simulink model "VisionModel_v6"  (Simulink 7.6)
settings: Solver=FixedStepDiscrete  StartTime=0.0  StopTime=0  RelTol=1e-3
values from neighbouring files (symbols this model uses):
  Iter_Segment_Thresh = 60    [VisionConstants.m]
  Scale_Down_B = 1    [VisionConstants.m]
  Scale_Down_G = 1    [VisionConstants.m]
  Scale_Down_H = 1    [VisionConstants.m]
  Scale_Down_R = 1    [VisionConstants.m]
  Scale_Down_S = 1    [VisionConstants.m]
  Scale_Down_V = 5    [VisionConstants.m]
  Scale_Forward_B = 0    [VisionConstants.m]
  Scale_Forward_G = 1    [VisionConstants.m]
  Scale_Forward_H = 1    [VisionConstants.m]
  Scale_Forward_R = 0    [VisionConstants.m]
  Scale_Forward_S = 1    [VisionConstants.m]
  Scale_Forward_V = 5    [VisionConstants.m]
undefined symbols (not defined in the file or in its folder): Rec, SDTV
libraries: vipconversions x4
settings Model: Creator=Administrator  LastModifiedBy=auvt
settings OptimizationCC: OptimizeModelRefInitCode=on
settings RTWCC: SystemTargetFile=ert.tlc  GenCodeOnly=on  TemplateMakefile=ert_default_tmf  PostCodeGenCommand=packNGo(buildInfo, {'packType' 'flat'})  Description=Real-Time Workshop Embedded Coder  GenerateReport=on  ProcessScript=ert_make_rtw_hook  IncludeHyperlinkInReport=on  LaunchReport=on  TargetLang=C++
settings CodeAppCC: IgnoreCustomStorageClasses=off
settings ERTTargetCC: MultiwordLength=2048  GenerateSampleERTMain=on  IncludeMdlTerminateFcn=off  ERTCustomFileTemplate=example_file_process.tlc  ConvertIfToSwitch=off

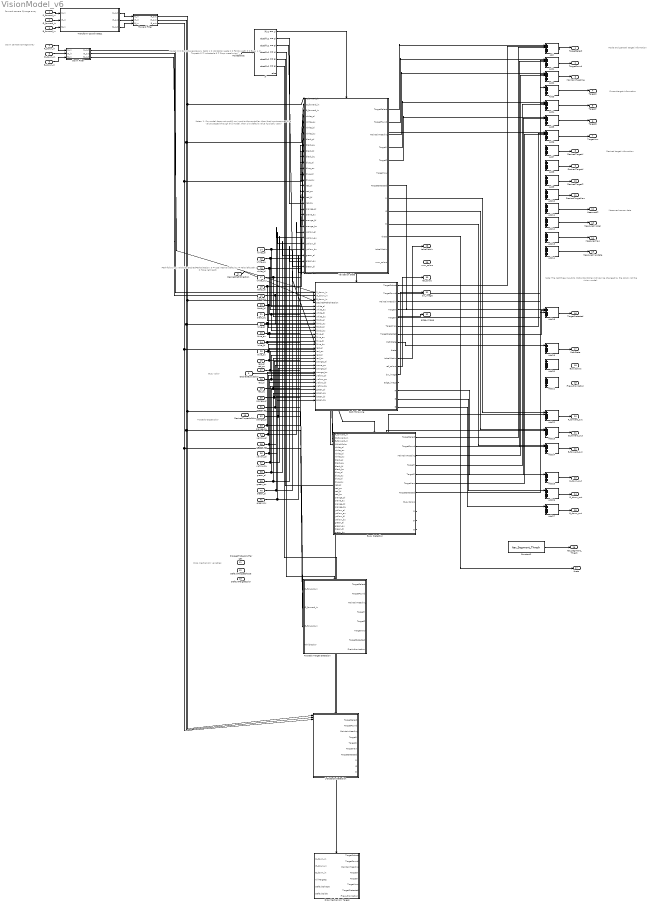
== system VisionModel_v6 ==
  note: Current target information
  note: Desired target information
  note: Measured sensor data
  note: Mode and general target information
  note: Forward camera QImage array
  note: Modes:
      | 0 = Do not execute any tasks
      | 1 = Validation gate
      | 2 = Follow path
      | 3 = Buoy
      | 4 = Torpedo
      | 5 = L-obstacle
      | 6 = Drop mecahnism
  note: Path-following variables
      | DesiredPathDirection:
      | 0 = Use internal default
      | 1 = Take left path
      | 2 = Take right path
  note: Buoy color
  note: Torpedo target color
  note: Drop mechanism variables
  note: Down camera QImage array
  note: Notes:
      | 1. If a model does not modify an input to the controller,
      | then that input assumes 1) a value passed through this
      | model, then 2) a default value (typically zero)
  note: Note: The last three inputs to MotionController.mdl
      | can be changed by the script, not the vision model.
  R_forward_in : Inport  PortDimensions=Forward_Camera_Dimensions
  G_forward_in : Inport  Port=2  PortDimensions=Forward_Camera_Dimensions
  B_forward_in : Inport  Port=3  PortDimensions=Forward_Camera_Dimensions
  R_down_in : Inport  Port=4  PortDimensions=Down_Camera_Dimensions
  G_down_in : Inport  Port=5  PortDimensions=Down_Camera_Dimensions
  B_down_in : Inport  Port=6  PortDimensions=Down_Camera_Dimensions
  ModeSelect : Inport  Port=7
  DesiredPathDirection : Inport  Port=8
  DesiredBuoyColor : Inport  Port=9
  DesiredTorpedoColor : Inport  Port=10
  ProceedToSecondTarget : Inport  Port=11
  DefaultTargetShape : Inport  Port=12
  DefaultTargetColor : Inport  Port=13
  white_al : Inport  Port=14
  white_au : Inport  Port=15
  white_bl : Inport  Port=16
  white_bu : Inport  Port=17
  black_al : Inport  Port=18
  black_au : Inport  Port=19
  black_bl : Inport  Port=20
  black_bu : Inport  Port=21
  blue_al : Inport  Port=22
  blue_au : Inport  Port=23
  blue_bl : Inport  Port=24
  blue_bu : Inport  Port=25
  red_al : Inport  Port=26
  red_au : Inport  Port=27
  red_bl : Inport  Port=28
  red_bu : Inport  Port=29
  orange_al : Inport  Port=30
  orane_au : Inport  Port=31
  orange_bl : Inport  Port=32
  orange_bu : Inport  Port=33
  yellow_al : Inport  Port=34
  yellow_au : Inport  Port=35
  yellow_bl : Inport  Port=36
  yellow_bu : Inport  Port=37
  green_al : Inport  Port=38
  green_au : Inport  Port=39
  breen_bl : Inport  Port=40
  green_bu : Inport  Port=41
  Add{,1..14,18..27} (25 alike) : Sum  Inputs=++++++
  Buoy Detection : Subsystem  TreatAsAtomicUnit=on
  Constant2 : Constant  Value=Iter_Segment_Thresh  SampleTime=-1
  Down Filter : Subsystem
  Drop Mechanism Target : Subsystem  TreatAsAtomicUnit=on
  Forward Filter : Subsystem
  If : If  IfExpression=u1 == 1  ElseIfExpressions=u1 == 2, u1 == 3, u1 == 4, u1 == 5, u1 == 6
  L-Obstacle Detection : Subsystem  TreatAsAtomicUnit=on
  Path Following : Subsystem  TreatAsAtomicUnit=on
  Torpedo Target Detection : Subsystem  TreatAsAtomicUnit=on
  Transform Coordinates1 : Stateflow chart  TreatAsAtomicUnit=on  SystemSampleTime=[1/30 0]
  Validation Gate : Subsystem  TreatAsAtomicUnit=on
  TargetSelect : Outport  OutDataTypeStr=double
  TargetFound : Outport  Port=2  OutDataTypeStr=double
  MaintainHeading : Outport  Port=3  OutDataTypeStr=double
  TargetX : Outport  Port=4  OutDataTypeStr=double
  TargetY : Outport  Port=5  OutDataTypeStr=double
  TargetZ : Outport  Port=6  OutDataTypeStr=double
  TargetYaw : Outport  Port=7  OutDataTypeStr=double
  DesiredTargetX : Outport  Port=8  OutDataTypeStr=double
  DesiredTargetY : Outport  Port=9  OutDataTypeStr=double
  DesiredTargetZ : Outport  Port=10  OutDataTypeStr=double
  DesiredTargetYaw : Outport  Port=11  OutDataTypeStr=double
  MeasuredZ : Outport  Port=12  OutDataTypeStr=double
  MeasuredYAccel : Outport  Port=13  OutDataTypeStr=double
  MeasuredYaw : Outport  Port=14  OutDataTypeStr=double
  MeasuredYawRate : Outport  Port=15  OutDataTypeStr=double
  TargetDetected : Outport  Port=16  OutDataTypeStr=double
  PathState : Outport  Port=17  OutDataTypeStr=double
  BuoyColors : Outport  Port=18  OutDataTypeStr=double
  FireAuthorization : Outport  Port=19  OutDataTypeStr=double
  R_forward_out : Outport  Port=20  OutDataTypeStr=double
  G_forward_out : Outport  Port=21  OutDataTypeStr=double
  B_forward_out : Outport  Port=22  OutDataTypeStr=double
  R_down_out : Outport  Port=23  OutDataTypeStr=double
  G_down_out : Outport  Port=24  OutDataTypeStr=double
  B_down_out : Outport  Port=25  OutDataTypeStr=double
  Iter_Segment_Thresh : Outport  Port=26  OutDataTypeStr=double
  theta : Outport  Port=27  OutDataTypeStr=double
  LabelMatrix : Outport  Port=28
  num_colors : Outport  Port=29
  ref_colors : Outport  Port=30
  bw_image : Outport  Port=31
  edge_image : Outport  Port=32
  wires:
  ModeSelect/1 -> If/1
  If/2 -> Path Following/Action
  If/3 -> Buoy Detection/Action
  If/1 -> Validation Gate/Action
  If/4 -> Torpedo Target Detection/Action
  If/5 -> L-Obstacle Detection/Action
  If/6 -> Drop Mechanism Target/Action
  DesiredBuoyColor/1 -> Buoy Detection/4(WhichColor)
  Down Filter/1(R_out) -> Path Following/1(R_down_in)
  Down Filter/2(G_out) -> Path Following/2(G_down_in)
  Down Filter/3(B_out) -> Path Following/3(B_down_in)
  Add/1 -> TargetSelect/1
  Add1/1 -> TargetFound/1
  Add2/1 -> MaintainHeading/1
  Add3/1 -> TargetX/1
  Add4/1 -> TargetY/1
  Add5/1 -> TargetZ/1
  Add6/1 -> TargetYaw/1
  Add7/1 -> DesiredTargetX/1
  Add8/1 -> DesiredTargetY/1
  Add9/1 -> DesiredTargetZ/1
  Add10/1 -> DesiredTargetYaw/1
  Add11/1 -> MeasuredZ/1
  Add12/1 -> MeasuredYAccel/1
  Add13/1 -> MeasuredYaw/1
  Add14/1 -> MeasuredYawRate/1
  Forward Filter/2(G_out) -> Validation Gate/2(G_forward_in), Buoy Detection/2(G_forward_in), Torpedo Target Detection/2(G_forward_in), L-Obstacle Detection/2(G_forward_in)
  Forward Filter/3(B_out) -> Validation Gate/3(B_forward_in), Buoy Detection/3(B_forward_in), Torpedo Target Detection/3(B_forward_in), L-Obstacle Detection/3(B_forward_in)
  Forward Filter/1(R_out) -> Validation Gate/1(R_forward_in), Buoy Detection/1(R_forward_in), Torpedo Target Detection/1(R_forward_in), L-Obstacle Detection/1(R_forward_in)
  G_down_in/1 -> Down Filter/2(G_in)
  R_down_in/1 -> Down Filter/1(R_in)
  B_down_in/1 -> Down Filter/3(B_in)
  Validation Gate/5(TargetZ) -> Add5/1
  Validation Gate/4(TargetY) -> Add4/1
  Validation Gate/1(TargetSelect) -> Add/1
  Validation Gate/2(TargetFound) -> Add1/1
  Validation Gate/3(MaintainHeading) -> Add2/1
  Validation Gate/6(TargetYaw) -> Add6/1
  Validation Gate/7(TargetDetected) -> Add18/1
  Add18/1 -> TargetDetected/1
  Constant2/1 -> Iter_Segment_Thresh/1
  Validation Gate/11(theta) -> theta/1
  G_forward_in/1 -> Transform Coordinates1/2(G_in)
  R_forward_in/1 -> Transform Coordinates1/1(R_in)
  B_forward_in/1 -> Transform Coordinates1/3(B_in)
  Transform Coordinates1/1(R_out) -> Forward Filter/1(R_in)
  Transform Coordinates1/2(G_out) -> Forward Filter/2(G_in)
  Transform Coordinates1/3(B_out) -> Forward Filter/3(B_in)
  Path Following/10(LabelMatrix) -> LabelMatrix/1
  ? -> num_colors/1
  Path Following/11(ref_colors) -> ref_colors/1
  Path Following/12(bw_image) -> bw_image/1
  Path Following/13(edge_image) -> edge_image/1
  Path Following/1(TargetSelect) -> Add/2
  Path Following/2(TargetFound) -> Add1/2
  Path Following/3(MaintainHeading) -> Add2/2
  Path Following/4(TargetX) -> Add3/1
  Path Following/5(TargetY) -> Add4/2
  Path Following/6(TargetYaw) -> Add6/2
  Path Following/7(TargetDetected) -> Add18/2
  Path Following/8(PathState) -> Add19/1
  Add19/1 -> PathState/1
  DesiredPathDirection/1 -> Path Following/4(DesiredPathDirection)
  Add22/1 -> R_forward_out/1
  Add23/1 -> G_forward_out/1
  Add24/1 -> B_forward_out/1
  Validation Gate/8(R) -> Add22/1
  Validation Gate/9(G) -> Add23/1
  Validation Gate/10(B) -> Add24/1
  Path Following/14(R) -> Add25/1
  Path Following/15(G) -> Add26/1
  Path Following/16(B) -> Add27/1
  Add25/1 -> R_down_out/1
  Add26/1 -> G_down_out/1
  Add27/1 -> B_down_out/1
  Buoy Detection/9(R) -> Add22/2
  Buoy Detection/10(G) -> Add23/2
  Buoy Detection/11(B) -> Add24/2
  Buoy Detection/1(TargetSelect) -> Add/3
  Buoy Detection/2(TargetFound) -> Add1/3
  Buoy Detection/3(MaintainHeading) -> Add2/3
  Buoy Detection/4(TargetY) -> Add4/3
  Buoy Detection/5(TargetZ) -> Add5/2
  Buoy Detection/6(TargetYaw) -> Add6/3
  Buoy Detection/7(TargetDetected) -> Add18/3
  white_al/1 -> Validation Gate/4(white_al), Path Following/5(white_al)
  white_au/1 -> Validation Gate/5(white_au), Path Following/6(white_au)
  white_bl/1 -> Validation Gate/6(white_bl), Path Following/7(white_bl)
  white_bu/1 -> Validation Gate/7(white_bu), Path Following/8(white_bu)
  black_al/1 -> Validation Gate/8(black_al), Path Following/9(black_al)
  black_au/1 -> Validation Gate/9(black_au), Path Following/10(black_au)
  black_bl/1 -> Validation Gate/10(black_bl), Path Following/11(black_bl)
  black_bu/1 -> Validation Gate/11(black_bu), Path Following/12(black_bu)
  blue_al/1 -> Validation Gate/12(blue_al), Path Following/13(blue_al)
  blue_au/1 -> Validation Gate/13(blue_au), Path Following/14(blue_au)
  blue_bl/1 -> Validation Gate/14(blue_bl), Path Following/15(blue_bl)
  blue_bu/1 -> Validation Gate/15(blue_bu), Path Following/16(blue_bu)
  red_al/1 -> Validation Gate/16(red_al), Path Following/17(red_al)
  red_au/1 -> Validation Gate/17(red_au), Path Following/18(red_au)
  red_bl/1 -> Validation Gate/18(red_bl), Path Following/19(red_bl)
  red_bu/1 -> Validation Gate/19(red_bu), Path Following/20(red_bu)
  orange_al/1 -> Validation Gate/20(orange_al), Path Following/21(orange_al)
  orane_au/1 -> Validation Gate/21(orane_au), Path Following/22(orane_au)
  orange_bl/1 -> Validation Gate/22(orange_bl), Path Following/23(orange_bl)
  orange_bu/1 -> Validation Gate/23(orange_bu), Path Following/24(orange_bu)
  yellow_al/1 -> Validation Gate/24(yellow_al), Path Following/25(yellow_al)
  yellow_au/1 -> Validation Gate/25(yellow_au), Path Following/26(yellow_au)
  yellow_bl/1 -> Validation Gate/26(yellow_bl), Path Following/27(yellow_bl)
  yellow_bu/1 -> Validation Gate/27(yellow_bu), Path Following/28(yellow_bu)
  green_al/1 -> Validation Gate/28(green_al), Path Following/29(green_al)
  green_au/1 -> Validation Gate/29(green_au), Path Following/30(green_au)
  breen_bl/1 -> Validation Gate/30(breen_bl), Path Following/31(breen_bl)
  green_bu/1 -> Validation Gate/31(green_bu), Path Following/32(green_bu)

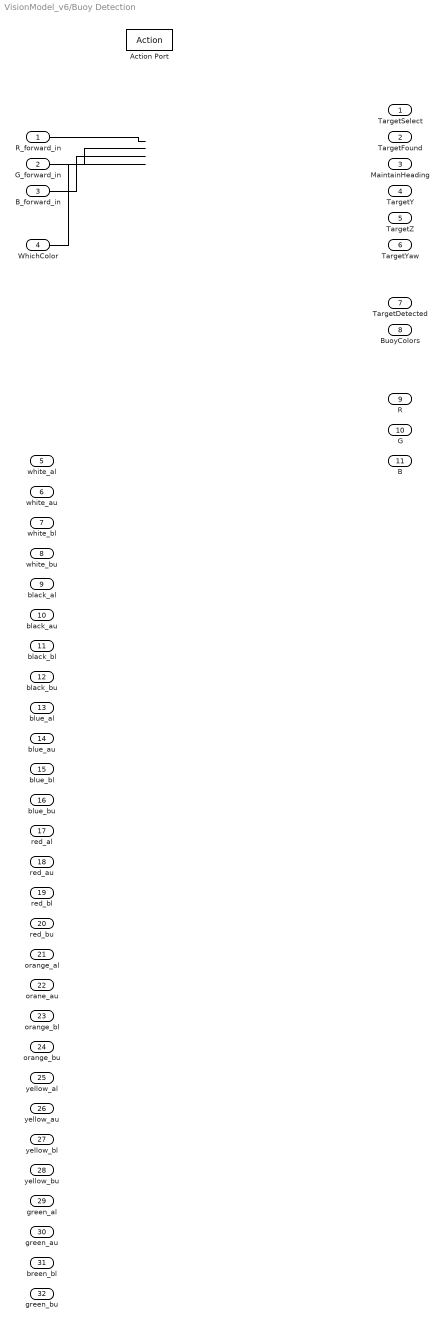
== system VisionModel_v6/Buoy Detection ==
  R_forward_in : Inport
  G_forward_in : Inport  Port=2
  B_forward_in : Inport  Port=3
  WhichColor : Inport  Port=4
  white_al : Inport  Port=5
  white_au : Inport  Port=6
  white_bl : Inport  Port=7
  white_bu : Inport  Port=8
  black_al : Inport  Port=9
  black_au : Inport  Port=10
  black_bl : Inport  Port=11
  black_bu : Inport  Port=12
  blue_al : Inport  Port=13
  blue_au : Inport  Port=14
  blue_bl : Inport  Port=15
  blue_bu : Inport  Port=16
  red_al : Inport  Port=17
  red_au : Inport  Port=18
  red_bl : Inport  Port=19
  red_bu : Inport  Port=20
  orange_al : Inport  Port=21
  orane_au : Inport  Port=22
  orange_bl : Inport  Port=23
  orange_bu : Inport  Port=24
  yellow_al : Inport  Port=25
  yellow_au : Inport  Port=26
  yellow_bl : Inport  Port=27
  yellow_bu : Inport  Port=28
  green_al : Inport  Port=29
  green_au : Inport  Port=30
  breen_bl : Inport  Port=31
  green_bu : Inport  Port=32
  Action Port : ActionPort  ActionType=elseif
  TargetSelect : Outport  OutDataTypeStr=double
  TargetFound : Outport  Port=2  OutDataTypeStr=double
  MaintainHeading : Outport  Port=3  OutDataTypeStr=double
  TargetY : Outport  Port=4  OutDataTypeStr=double
  TargetZ : Outport  Port=5  OutDataTypeStr=double
  TargetYaw : Outport  Port=6  OutDataTypeStr=double
  TargetDetected : Outport  Port=7  OutDataTypeStr=double
  BuoyColors : Outport  Port=8  OutDataTypeStr=double
  R : Outport  Port=9  OutDataTypeStr=double
  G : Outport  Port=10  OutDataTypeStr=double
  B : Outport  Port=11  OutDataTypeStr=double
  wires:
  R_forward_in/1 -> ?
  G_forward_in/1 -> ?
  B_forward_in/1 -> ?
  WhichColor/1 -> ?
  ? -> TargetSelect/1
  ? -> TargetFound/1
  ? -> MaintainHeading/1
  ? -> TargetY/1
  ? -> TargetZ/1
  ? -> TargetYaw/1
  ? -> TargetDetected/1
  ? -> BuoyColors/1
  ? -> R/1
  ? -> G/1
  ? -> B/1

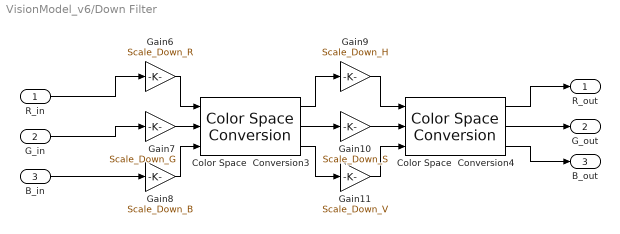
== system VisionModel_v6/Down Filter ==
  R_in : Inport  PortDimensions=Down_Camera_Dimensions
  G_in : Inport  Port=2  PortDimensions=Down_Camera_Dimensions
  B_in : Inport  Port=3  PortDimensions=Down_Camera_Dimensions
  Color Space  Conversion3 : vipconversions/Color Space  Conversion  conversion=Obsolete  conversionActive=R'G'B' to HSV  wp_str=D50  rec=Rec. 601 (SDTV)  sys=1125/60/2:1  imagePorts=Separate color signals
  Color Space  Conversion4 : vipconversions/Color Space  Conversion  conversion=Obsolete  conversionActive=HSV to R'G'B'  wp_str=D50  rec=Rec. 601 (SDTV)  sys=1125/60/2:1  imagePorts=Separate color signals
  Gain10 : Gain  Gain=Scale_Down_S
  Gain11 : Gain  Gain=Scale_Down_V
  Gain6 : Gain  Gain=Scale_Down_R
  Gain7 : Gain  Gain=Scale_Down_G
  Gain8 : Gain  Gain=Scale_Down_B
  Gain9 : Gain  Gain=Scale_Down_H
  R_out : Outport  OutDataTypeStr=double
  G_out : Outport  Port=2  OutDataTypeStr=double
  B_out : Outport  Port=3  OutDataTypeStr=double
  wires:
  Gain6/1 -> Color Space  Conversion3/1
  Gain7/1 -> Color Space  Conversion3/2
  Gain8/1 -> Color Space  Conversion3/3
  Color Space  Conversion3/1 -> Gain9/1
  Color Space  Conversion3/2 -> Gain10/1
  Color Space  Conversion3/3 -> Gain11/1
  Gain9/1 -> Color Space  Conversion4/1
  Gain10/1 -> Color Space  Conversion4/2
  Gain11/1 -> Color Space  Conversion4/3
  R_in/1 -> Gain6/1
  G_in/1 -> Gain7/1
  B_in/1 -> Gain8/1
  Color Space  Conversion4/1 -> R_out/1
  Color Space  Conversion4/2 -> G_out/1
  Color Space  Conversion4/3 -> B_out/1

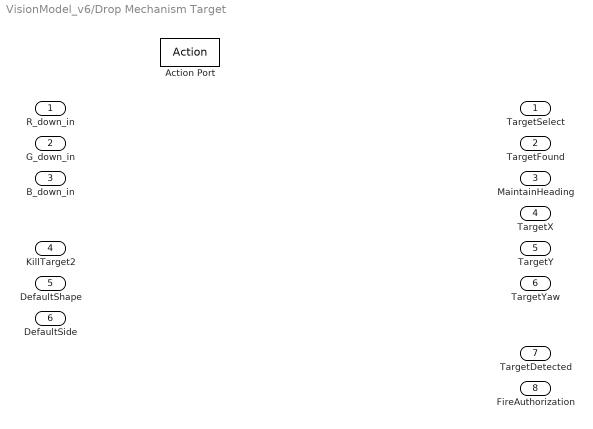
== system VisionModel_v6/Drop Mechanism Target ==
  R_down_in : Inport
  G_down_in : Inport  Port=2
  B_down_in : Inport  Port=3
  KillTarget2 : Inport  Port=4
  DefaultShape : Inport  Port=5
  DefaultSide : Inport  Port=6
  Action Port : ActionPort  ActionType=elseif
  TargetSelect : Outport  OutDataTypeStr=double
  TargetFound : Outport  Port=2  OutDataTypeStr=double
  MaintainHeading : Outport  Port=3  OutDataTypeStr=double
  TargetX : Outport  Port=4  OutDataTypeStr=double
  TargetY : Outport  Port=5  OutDataTypeStr=double
  TargetYaw : Outport  Port=6  OutDataTypeStr=double
  TargetDetected : Outport  Port=7  OutDataTypeStr=double
  FireAuthorization : Outport  Port=8  OutDataTypeStr=double

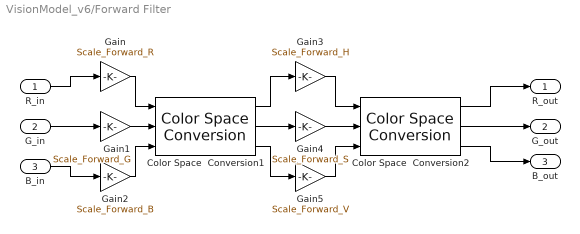
== system VisionModel_v6/Forward Filter ==
  R_in : Inport  PortDimensions=Forward_Camera_Dimensions
  G_in : Inport  Port=2  PortDimensions=Forward_Camera_Dimensions
  B_in : Inport  Port=3  PortDimensions=Forward_Camera_Dimensions
  Color Space  Conversion1 : vipconversions/Color Space  Conversion  conversion=Obsolete  conversionActive=R'G'B' to HSV  wp_str=D50  rec=Rec. 601 (SDTV)  sys=1125/60/2:1  imagePorts=Separate color signals
  Color Space  Conversion2 : vipconversions/Color Space  Conversion  conversion=Obsolete  conversionActive=HSV to R'G'B'  wp_str=D50  rec=Rec. 601 (SDTV)  sys=1125/60/2:1  imagePorts=Separate color signals
  Gain : Gain  Gain=Scale_Forward_R
  Gain1 : Gain  Gain=Scale_Forward_G
  Gain2 : Gain  Gain=Scale_Forward_B
  Gain3 : Gain  Gain=Scale_Forward_H
  Gain4 : Gain  Gain=Scale_Forward_S
  Gain5 : Gain  Gain=Scale_Forward_V
  R_out : Outport  OutDataTypeStr=double
  G_out : Outport  Port=2  OutDataTypeStr=double
  B_out : Outport  Port=3  OutDataTypeStr=double
  wires:
  R_in/1 -> Gain/1
  G_in/1 -> Gain1/1
  B_in/1 -> Gain2/1
  Gain/1 -> Color Space  Conversion1/1
  Gain1/1 -> Color Space  Conversion1/2
  Gain2/1 -> Color Space  Conversion1/3
  Color Space  Conversion1/1 -> Gain3/1
  Color Space  Conversion1/2 -> Gain4/1
  Color Space  Conversion1/3 -> Gain5/1
  Gain3/1 -> Color Space  Conversion2/1
  Gain4/1 -> Color Space  Conversion2/2
  Gain5/1 -> Color Space  Conversion2/3
  Color Space  Conversion2/1 -> R_out/1
  Color Space  Conversion2/2 -> G_out/1
  Color Space  Conversion2/3 -> B_out/1

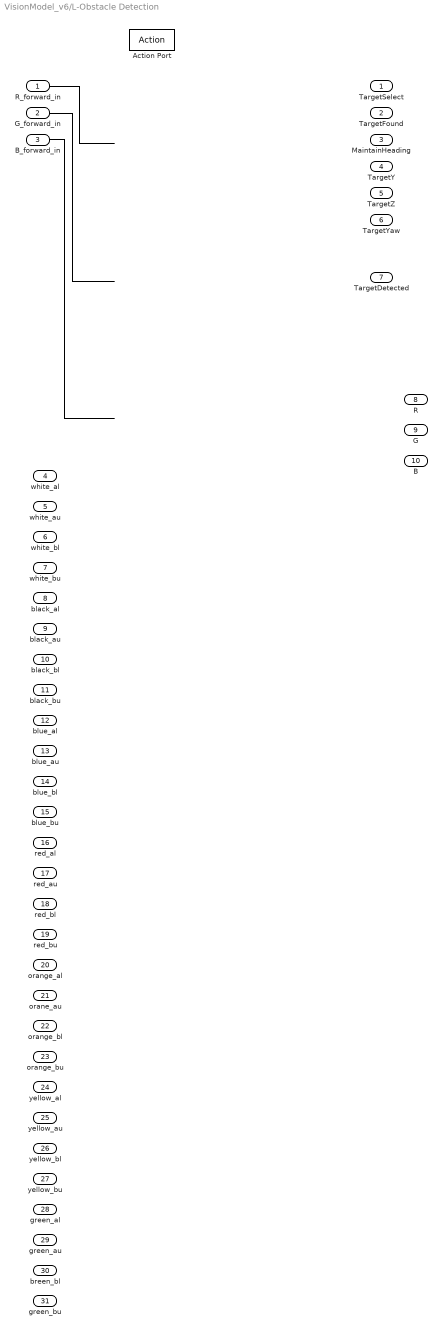
== system VisionModel_v6/L-Obstacle Detection ==
  R_forward_in : Inport
  G_forward_in : Inport  Port=2
  B_forward_in : Inport  Port=3
  white_al : Inport  Port=4
  white_au : Inport  Port=5
  white_bl : Inport  Port=6
  white_bu : Inport  Port=7
  black_al : Inport  Port=8
  black_au : Inport  Port=9
  black_bl : Inport  Port=10
  black_bu : Inport  Port=11
  blue_al : Inport  Port=12
  blue_au : Inport  Port=13
  blue_bl : Inport  Port=14
  blue_bu : Inport  Port=15
  red_al : Inport  Port=16
  red_au : Inport  Port=17
  red_bl : Inport  Port=18
  red_bu : Inport  Port=19
  orange_al : Inport  Port=20
  orane_au : Inport  Port=21
  orange_bl : Inport  Port=22
  orange_bu : Inport  Port=23
  yellow_al : Inport  Port=24
  yellow_au : Inport  Port=25
  yellow_bl : Inport  Port=26
  yellow_bu : Inport  Port=27
  green_al : Inport  Port=28
  green_au : Inport  Port=29
  breen_bl : Inport  Port=30
  green_bu : Inport  Port=31
  Action Port : ActionPort  ActionType=elseif
  TargetSelect : Outport  OutDataTypeStr=double
  TargetFound : Outport  Port=2  OutDataTypeStr=double
  MaintainHeading : Outport  Port=3  OutDataTypeStr=double
  TargetY : Outport  Port=4  OutDataTypeStr=double
  TargetZ : Outport  Port=5  OutDataTypeStr=double
  TargetYaw : Outport  Port=6  OutDataTypeStr=double
  TargetDetected : Outport  Port=7  OutDataTypeStr=double
  R : Outport  Port=8  OutDataTypeStr=double
  G : Outport  Port=9  OutDataTypeStr=double
  B : Outport  Port=10  OutDataTypeStr=double
  wires:
  R_forward_in/1 -> ?
  G_forward_in/1 -> ?
  B_forward_in/1 -> ?
  ? -> TargetSelect/1
  ? -> TargetFound/1
  ? -> MaintainHeading/1
  ? -> TargetY/1
  ? -> TargetZ/1
  ? -> TargetYaw/1
  ? -> TargetDetected/1
  ? -> R/1
  ? -> G/1
  ? -> B/1

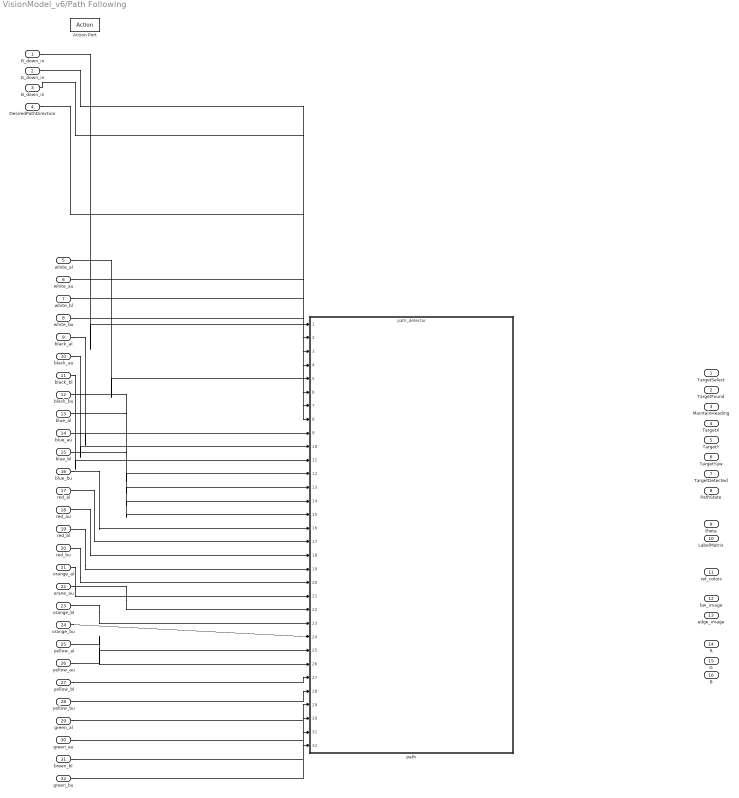
== system VisionModel_v6/Path Following ==
  R_down_in : Inport
  G_down_in : Inport  Port=2
  B_down_in : Inport  Port=3
  DesiredPathDirection : Inport  Port=4
  white_al : Inport  Port=5
  white_au : Inport  Port=6
  white_bl : Inport  Port=7
  white_bu : Inport  Port=8
  black_al : Inport  Port=9
  black_au : Inport  Port=10
  black_bl : Inport  Port=11
  black_bu : Inport  Port=12
  blue_al : Inport  Port=13
  blue_au : Inport  Port=14
  blue_bl : Inport  Port=15
  blue_bu : Inport  Port=16
  red_al : Inport  Port=17
  red_au : Inport  Port=18
  red_bl : Inport  Port=19
  red_bu : Inport  Port=20
  orange_al : Inport  Port=21
  orane_au : Inport  Port=22
  orange_bl : Inport  Port=23
  orange_bu : Inport  Port=24
  yellow_al : Inport  Port=25
  yellow_au : Inport  Port=26
  yellow_bl : Inport  Port=27
  yellow_bu : Inport  Port=28
  green_al : Inport  Port=29
  green_au : Inport  Port=30
  breen_bl : Inport  Port=31
  green_bu : Inport  Port=32
  Action Port : ActionPort  ActionType=elseif
  path : ModelReference  ModelNameDialog=path_detector  SimulationMode=Accelerator  ModelReferenceVersion=1.402  CopyOfModelName=path_detector
  TargetSelect : Outport  OutDataTypeStr=double
  TargetFound : Outport  Port=2  OutDataTypeStr=double
  MaintainHeading : Outport  Port=3  OutDataTypeStr=double
  TargetX : Outport  Port=4  OutDataTypeStr=double
  TargetY : Outport  Port=5  OutDataTypeStr=double
  TargetYaw : Outport  Port=6  OutDataTypeStr=double
  TargetDetected : Outport  Port=7  OutDataTypeStr=double
  PathState : Outport  Port=8  OutDataTypeStr=double
  theta : Outport  Port=9  OutDataTypeStr=double
  LabelMatrix : Outport  Port=10
  ref_colors : Outport  Port=11
  bw_image : Outport  Port=12
  edge_image : Outport  Port=13
  R : Outport  Port=14  OutDataTypeStr=double
  G : Outport  Port=15  OutDataTypeStr=double
  B : Outport  Port=16  OutDataTypeStr=double
  wires:
  R_down_in/1 -> path/1
  G_down_in/1 -> path/2
  B_down_in/1 -> path/3
  DesiredPathDirection/1 -> path/4
  white_al/1 -> path/5
  white_au/1 -> path/6
  white_bl/1 -> path/7
  white_bu/1 -> path/8
  black_al/1 -> path/9
  black_au/1 -> path/10
  black_bl/1 -> path/11
  black_bu/1 -> path/12
  blue_al/1 -> path/13
  blue_au/1 -> path/14
  blue_bl/1 -> path/15
  blue_bu/1 -> path/16
  red_al/1 -> path/17
  red_au/1 -> path/18
  red_bl/1 -> path/19
  red_bu/1 -> path/20
  orange_al/1 -> path/21
  orane_au/1 -> path/22
  orange_bl/1 -> path/23
  orange_bu/1 -> path/24
  yellow_al/1 -> path/25
  yellow_au/1 -> path/26
  yellow_bl/1 -> path/27
  yellow_bu/1 -> path/28
  green_al/1 -> path/29
  green_au/1 -> path/30
  breen_bl/1 -> path/31
  green_bu/1 -> path/32
  ? -> TargetSelect/1
  ? -> TargetFound/1
  ? -> MaintainHeading/1
  ? -> TargetX/1
  ? -> TargetY/1
  ? -> TargetYaw/1
  ? -> TargetDetected/1
  ? -> PathState/1
  ? -> R/1
  ? -> G/1
  ? -> B/1

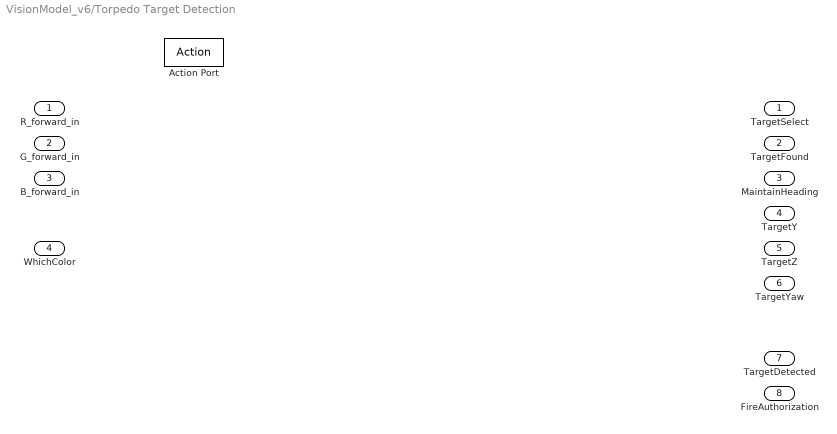
== system VisionModel_v6/Torpedo Target Detection ==
  R_forward_in : Inport
  G_forward_in : Inport  Port=2
  B_forward_in : Inport  Port=3
  WhichColor : Inport  Port=4
  Action Port : ActionPort  ActionType=elseif
  TargetSelect : Outport  OutDataTypeStr=double
  TargetFound : Outport  Port=2  OutDataTypeStr=double
  MaintainHeading : Outport  Port=3  OutDataTypeStr=double
  TargetY : Outport  Port=4  OutDataTypeStr=double
  TargetZ : Outport  Port=5  OutDataTypeStr=double
  TargetYaw : Outport  Port=6  OutDataTypeStr=double
  TargetDetected : Outport  Port=7  OutDataTypeStr=double
  FireAuthorization : Outport  Port=8  OutDataTypeStr=double

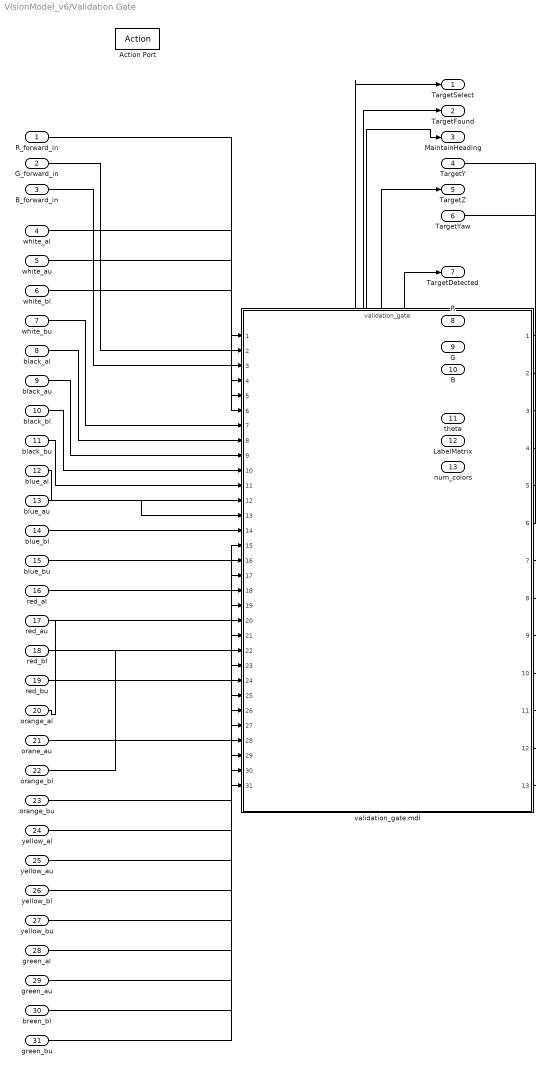
== system VisionModel_v6/Validation Gate ==
  R_forward_in : Inport
  G_forward_in : Inport  Port=2
  B_forward_in : Inport  Port=3
  white_al : Inport  Port=4
  white_au : Inport  Port=5
  white_bl : Inport  Port=6
  white_bu : Inport  Port=7
  black_al : Inport  Port=8
  black_au : Inport  Port=9
  black_bl : Inport  Port=10
  black_bu : Inport  Port=11
  blue_al : Inport  Port=12
  blue_au : Inport  Port=13
  blue_bl : Inport  Port=14
  blue_bu : Inport  Port=15
  red_al : Inport  Port=16
  red_au : Inport  Port=17
  red_bl : Inport  Port=18
  red_bu : Inport  Port=19
  orange_al : Inport  Port=20
  orane_au : Inport  Port=21
  orange_bl : Inport  Port=22
  orange_bu : Inport  Port=23
  yellow_al : Inport  Port=24
  yellow_au : Inport  Port=25
  yellow_bl : Inport  Port=26
  yellow_bu : Inport  Port=27
  green_al : Inport  Port=28
  green_au : Inport  Port=29
  breen_bl : Inport  Port=30
  green_bu : Inport  Port=31
  Action Port : ActionPort  ActionType=then
  validation_gate.mdl : ModelReference  ModelNameDialog=validation_gate  SimulationMode=Accelerator  ModelReferenceVersion=1.1298  CopyOfModelName=validation_gate
  TargetSelect : Outport  OutDataTypeStr=double
  TargetFound : Outport  Port=2  OutDataTypeStr=double
  MaintainHeading : Outport  Port=3  OutDataTypeStr=double
  TargetY : Outport  Port=4  OutDataTypeStr=double
  TargetZ : Outport  Port=5  OutDataTypeStr=double
  TargetYaw : Outport  Port=6  OutDataTypeStr=double
  TargetDetected : Outport  Port=7  OutDataTypeStr=double
  R : Outport  Port=8  OutDataTypeStr=double
  G : Outport  Port=9  OutDataTypeStr=double
  B : Outport  Port=10  OutDataTypeStr=double
  theta : Outport  Port=11  OutDataTypeStr=double
  LabelMatrix : Outport  Port=12
  num_colors : Outport  Port=13
  wires:
  R_forward_in/1 -> validation_gate.mdl/1
  G_forward_in/1 -> validation_gate.mdl/2
  B_forward_in/1 -> validation_gate.mdl/3
  validation_gate.mdl/7 -> TargetDetected/1
  validation_gate.mdl/4 -> TargetY/1
  validation_gate.mdl/5 -> TargetZ/1
  validation_gate.mdl/1 -> TargetSelect/1
  validation_gate.mdl/2 -> TargetFound/1
  validation_gate.mdl/3 -> MaintainHeading/1
  validation_gate.mdl/6 -> TargetYaw/1
  validation_gate.mdl/8 -> R/1
  validation_gate.mdl/9 -> G/1
  validation_gate.mdl/10 -> B/1
  validation_gate.mdl/11 -> theta/1
  validation_gate.mdl/12 -> LabelMatrix/1
  validation_gate.mdl/13 -> num_colors/1
  white_al/1 -> validation_gate.mdl/4
  white_au/1 -> validation_gate.mdl/5
  white_bl/1 -> validation_gate.mdl/6
  white_bu/1 -> validation_gate.mdl/7
  black_al/1 -> validation_gate.mdl/8
  black_au/1 -> validation_gate.mdl/9
  black_bl/1 -> validation_gate.mdl/10
  black_bu/1 -> validation_gate.mdl/11
  blue_al/1 -> validation_gate.mdl/12
  blue_au/1 -> validation_gate.mdl/13
  blue_bl/1 -> validation_gate.mdl/14
  blue_bu/1 -> validation_gate.mdl/15
  red_al/1 -> validation_gate.mdl/16
  red_au/1 -> validation_gate.mdl/17
  red_bl/1 -> validation_gate.mdl/18
  red_bu/1 -> validation_gate.mdl/19
  orange_al/1 -> validation_gate.mdl/20
  orane_au/1 -> validation_gate.mdl/21
  orange_bl/1 -> validation_gate.mdl/22
  orange_bu/1 -> validation_gate.mdl/23
  yellow_al/1 -> validation_gate.mdl/24
  yellow_au/1 -> validation_gate.mdl/25
  yellow_bl/1 -> validation_gate.mdl/26
  yellow_bu/1 -> validation_gate.mdl/27
  green_al/1 -> validation_gate.mdl/28
  green_au/1 -> validation_gate.mdl/29
  breen_bl/1 -> validation_gate.mdl/30
  green_bu/1 -> validation_gate.mdl/31

== matlab function Transform Coordinates1 ==
  data: R_in input double; G_in input double; R_out output double; G_out output double; B_in input double; B_out output double
function [R_out, G_out, B_out] = rangeImage(R_in, G_in, B_in)
unction [R_out, G_out, B_out] = rangeImage(R_in, G_in, B_in)
% Ensure the image components are between 0 and newMax

newMax = 1;

R_out = R_in;
G_out = G_in;
B_out = B_in;

normalizeValue = max(max(R_in));
if( normalizeValue <= 1 )
    normalizeValue = 1;
else
    normalizeValue = 255;
end

[rows, cols] = size(R_in);


for r = 1:rows
    for c = 1:cols
        
        if( R_in(r,c) == 0 )
            R_out(r,c) = 0;
        else
            R_out(r,c) = newMax*R_in(r,c)/normalizeValue;
        end
        if( G_in(r,c) == 0 )
            G_out(r,c) = 0;
        else
            G_out(r,c) = newMax*G_in(r,c)/normalizeValue;
        end
        if( B_in(r,c) == 0 )
            B_out(r,c) = 0;
        else
            B_out(r,c) = newMax*B_in(r,c)/normalizeValue;
        end
        
    end
end


return
